simulink model "deadbeat_running_control"  (R2016b)
settings: configuration reference "Configuration1khz" (kept outside this file)
undefined symbols (not defined in the file or in its folder): A_kalman_no_position, A_kalman_transverse, A_kalman_vertical, A_lpf_accelerometer, A_lpf_contact, A_lpf_imu, A_lpf_lateral_angle, B1_lpf_accelerometer, B1_lpf_contact, B1_lpf_imu, B1_lpf_lateral_angle, B2_lpf_accelerometer, B2_lpf_contact, B2_lpf_imu, B2_lpf_lateral_angle, B_dx_versus_x0, B_kalman_no_position, B_kalman_transverse, B_kalman_vertical, backwards_K_sag_of_t, backwards_P_sag_of_t, C_kalman_no_position, C_kalman_transverse, C_kalman_vertical, com_leg_motor, com_torso, contact_threshold, d_ankle_to_foot, d_vertical_com, desired_com_forward_velocity, desired_com_lateral_velocity, desired_standing_torso_pitch, desired_standing_torso_roll, desired_standing_z, desired_torso_pitch, desired_torso_roll, DiscIntNeverNeededParam, Discrete, enable_bouncing, fdesignblkfcn, flight_duration, forward_dx_of_dxstar, forward_x_of_dxstar, g, gcbh, HIP_MTR_MAX_CONT_TORQUE, HIP_MTR_MAX_TORQUE, i_leg_motor, i_robot, i_torso, initial_dx_estimate, initial_dx_takeoff_history, initial_dx_touchdown_history, initial_dy_estimate, initial_dy_takeoff_history, initial_dy_touchdown_history, initial_dz_estimate, initial_leg_selection, initial_target_dx_history, initial_target_dy_history ... (+80)
libraries: simulink x22, ctrlSharedLib x4, dsparch4 x2
(part 5 of 7)

== matlab function deadbeat_running_control/Behavior/Primary and Lateral Behavior/Circular Buffer (Right Foot)/Buffer1 ==
  data: initial_data input; data input; buffer output size=recorded_steps; trigger input; buffer_size input
function buffer  = buffer_data(initial_data, data, trigger, buffer_size)

    persistent buffer_memory
    coder.varsize('buffer_memory',500);
    if isempty(buffer_memory)
        buffer_memory = initial_data;
        if isnan(initial_data(1))
            buffer_memory = [];
        end
    end
    
    if trigger
        buffer_memory = [data; buffer_memory];
        if size(buffer_memory, 1) > buffer_size
            buffer_memory = buffer_memory(1:buffer_size,:);
        end
    end
    
    buffer = buffer_memory;

end

== matlab function deadbeat_running_control/Behavior/Primary and Lateral Behavior/Circular Buffer (Right Foot)/Buffer2 ==
  data: initial_data input; data input; buffer output size=recorded_steps; trigger input; buffer_size input
function buffer  = buffer_data(initial_data, data, trigger, buffer_size)

    persistent buffer_memory
    coder.varsize('buffer_memory',500);
    if isempty(buffer_memory)
        buffer_memory = initial_data;
        if isnan(initial_data(1))
            buffer_memory = [];
        end
    end
    
    if trigger
        buffer_memory = [data; buffer_memory];
        if size(buffer_memory, 1) > buffer_size
            buffer_memory = buffer_memory(1:buffer_size,:);
        end
    end
    
    buffer = buffer_memory;

end

== matlab function deadbeat_running_control/Behavior/Atrias Swing control/Avoid Hitting Mechanical Limits ==
  data: back_cmd output double; front_cmd output double; dback_cmd output double; dfront_cmd output double; ddback_cmd output double; ddfront_cmd output double; back_desired input; dback_desired input; ddback_desired input; front_desired input; dfront_desired input; ddfront_desired input; min_front_bar_angle parameter; max_front_bar_angle parameter; min_back_bar_angle parameter; max_back_bar_angle parameter
%% Avoid joint limits by ensuring we don't command velocities/accelerations that would push us into them when we are close to them.
function [back_cmd, front_cmd, dback_cmd, dfront_cmd, ddback_cmd, ddfront_cmd] ...
    = AvoidFourbarLimits(back_desired,dback_desired, ddback_desired, ...
          front_desired, dfront_desired, ddfront_desired, ...
          min_front_bar_angle, max_front_bar_angle, min_back_bar_angle, max_back_bar_angle)
    [back_cmd, front_cmd, dback_cmd, dfront_cmd, ddback_cmd, ddfront_cmd] = AvoidFourbarLimits(back_desired,dback_desired, ddback_desired, front_desired, dfront_desired, ddfront_desired, min_front_bar_angle, max_front_bar_angle, min_back_bar_angle, max_back_bar_angle);
end

== matlab function deadbeat_running_control/Behavior/Atrias Swing control/Convert COM Position to Joint Angles + Leg Length  ==
  data: desired_leg_length output; X_star input; Y_star input; Z_star input; right_left input; com_pelvis_body input; desired_alpha output; desired_beta output; dcom_pelvis_body input; roll input; pitch input; sagittal_angle input; lateral_angle input; leg_length input; lateral_offset parameter; minimum_lateral_beta parameter; maximum_lateral_beta parameter
function [ desired_leg_length, desired_alpha, desired_beta ]  =  ...
          ConvertToJointAnglesAndLegLength(X_star, Y_star, Z_star, right_left,...
                           com_pelvis_body, dcom_pelvis_body, ...
                           roll, pitch, sagittal_angle, lateral_angle, leg_length,...
                           lateral_offset, minimum_lateral_beta, maximum_lateral_beta) 

    q = [roll(1), pitch(1), sagittal_angle(1), lateral_angle(1), leg_length(1)];
    dq = [roll(2), pitch(2), sagittal_angle(2), lateral_angle(2), leg_length(2)];
    [desired_alpha, desired_beta, desired_leg_length]  =  ConvertComPositionToLegAnglesAndLegLength(X_star, Y_star, Z_star, right_left, com_pelvis_body, dcom_pelvis_body, q, dq, lateral_offset);   
    desired_beta = saturate(desired_beta, minimum_lateral_beta, maximum_lateral_beta);
end

function [desired_saturated] = saturate(desired, minimum_lateral_beta, maximum_lateral_beta)
    desired_saturated = desired;
    if desired(1) < minimum_lateral_beta
        desired_saturated = [minimum_lateral_beta; 0; 0];
    elseif desired(1) > maximum_lateral_beta
        desired_saturated = [maximum_lateral_beta; 0; 0];    
    end
end

== matlab function deadbeat_running_control/Behavior/Atrias Swing control/Virtual Leg to Four Bar ==
  data: l_leg input; dl_leg input; ddl_leg input; phi input; dphi input; ddphi input; back output; dback output; ddback output; front output; dfront output; ddfront output
function [back, dback, ddback, front, dfront, ddfront] = VirtualLegToFourBar(l_leg, dl_leg, ddl_leg, phi, dphi, ddphi)
    [back, dback, ddback, front, dfront, ddfront] = VirtualLegToFourBar(l_leg, dl_leg, ddl_leg, phi, dphi, ddphi);
end

== matlab function deadbeat_running_control/Behavior/Primary and Lateral Behavior/Circular Buffer (Right Foot)/Buffer3 ==
  data: initial_data input; data input; buffer output size=recorded_steps; trigger input; buffer_size input
function buffer  = buffer_data(initial_data, data, trigger, buffer_size)

    persistent buffer_memory
    coder.varsize('buffer_memory',500);
    if isempty(buffer_memory)
        buffer_memory = initial_data;
        if isnan(initial_data(1))
            buffer_memory = [];
        end
    end
    
    if trigger
        buffer_memory = [data; buffer_memory];
        if size(buffer_memory, 1) > buffer_size
            buffer_memory = buffer_memory(1:buffer_size,:);
        end
    end
    
    buffer = buffer_memory;

end

== matlab function deadbeat_running_control/Behavior/Primary and Lateral Behavior/Circular Buffer (Right Foot)/Buffer4 ==
  data: initial_data input; data input; buffer output size=recorded_steps; trigger input; buffer_size input
function buffer  = buffer_data(initial_data, data, trigger, buffer_size)

    persistent buffer_memory
    coder.varsize('buffer_memory',500);
    if isempty(buffer_memory)
        buffer_memory = initial_data;
        if isnan(initial_data(1))
            buffer_memory = [];
        end
    end
    
    if trigger
        buffer_memory = [data; buffer_memory];
        if size(buffer_memory, 1) > buffer_size
            buffer_memory = buffer_memory(1:buffer_size,:);
        end
    end
    
    buffer = buffer_memory;

end

== stateflow chart deadbeat_running_control/Behavior/Contact State Machine/State Machine ==
  state Touchdown
  state Unloading
  state Takeoff
  state Flight
  Touchdown -> (junction 162) [order 2] : [contact_factor < 0.5*contact_threshold]
  (junction 162) -> (junction 128)
  (junction 115) -> Touchdown
  (junction 118) -> (junction 115)
  Touchdown -> Unloading [order 1] : [z_velocity >= 0 && previous_z_velocity < 0]
  Unloading -> Touchdown [order 2] : [contact_factor > contact_threshold && z_velocity < 0]
  (junction 122) -> (junction 118)
  Unloading -> Takeoff [order 1] : [contact_factor < contact_threshold]
  (junction 172) -> (junction 122)
  Takeoff -> Flight : after(t_flight,sec)
  (default) -> Flight
  Flight -> (junction 172) : [contact_factor > variable_contact_threshold]
  (junction 128) -> Flight
  data: z_velocity input; previous_z_velocity input; contact_factor input; t_flight parameter; contact_threshold parameter; Touchdown output boolean; Unloading output boolean; Takeoff output boolean; Flight output boolean; variable_contact_threshold input

== matlab function deadbeat_running_control/Behavior/Primary and Lateral Behavior/Circular Buffer (Right Foot)/Buffer6 ==
  data: initial_data input; data input; buffer output size=recorded_steps; trigger input; buffer_size input
function buffer  = buffer_data(initial_data, data, trigger, buffer_size)

    persistent buffer_memory
    coder.varsize('buffer_memory',500);
    if isempty(buffer_memory)
        buffer_memory = initial_data;
        if isnan(initial_data(1))
            buffer_memory = [];
        end
    end
    
    if trigger
        buffer_memory = [data; buffer_memory];
        if size(buffer_memory, 1) > buffer_size
            buffer_memory = buffer_memory(1:buffer_size,:);
        end
    end
    
    buffer = buffer_memory;

end

== matlab function deadbeat_running_control/Behavior/Force Estimation/3D Forward Dynamics yawed ==
  data: right_or_left input; torso_roll input size=2; torso_pitch input double size=2; torso_yaw input double size=2; primary_sagittal_leg_angle input double size=2; primary_leg_length input double size=2; primary_leg_roll input double size=2; secondary_leg_roll input double size=2; primary_leg_torque input; primary_leg_force input; primary_lateral_torque input; secondary_lateral_torque input; R_GRF output double size=3; L_GRF output size=3; ddroll output double; g parameter; m_leg_motor parameter; m_torso parameter; i_torso parameter; i_leg_motor parameter; lateral_offset parameter; com_torso parameter; torso_centerline_roll_offset_angle parameter
%% Forward 3D ATRIAS dynamics
function [R_GRF, L_GRF, ddroll]  =  ForwardDynamics3D(right_or_left, ...
                                                      torso_roll, torso_pitch, torso_yaw, ...
                                                      primary_sagittal_leg_angle, primary_leg_length,...
                                                      primary_leg_roll, secondary_leg_roll, ...
                                                      primary_leg_torque, primary_leg_force, ...
                                                      primary_lateral_torque, secondary_lateral_torque, ...
                                                      g, m_leg_motor, m_torso, i_torso, i_leg_motor, lateral_offset, com_torso, torso_centerline_roll_offset_angle)

    d = norm(com_torso(2:3));
    It = mean(i_torso);
    Im = mean(i_leg_motor);
    
    phi    = torso_roll(1) + torso_centerline_roll_offset_angle;  % roll
    theta  = torso_pitch(1);                   % pitch
    alpha1 = primary_sagittal_leg_angle(1);    % primary sagittal leg angle
    beta1  = primary_leg_roll(1);              % primary leg roll
    beta2  = secondary_leg_roll(1);            % secondary leg roll
    if right_or_left
        beta1 = beta1 - torso_centerline_roll_offset_angle;
        beta2 = beta2 + torso_centerline_roll_offset_angle;
    else
        beta1 = beta1 + torso_centerline_roll_offset_angle;
        beta2 = beta2 - torso_centerline_roll_offset_angle;
    end 
    l1     = primary_leg_length(1);            % primary leg length
    
    dphi    = torso_roll(2);
    dtheta  = torso_pitch(2);
    dpsi    = torso_yaw(2);
    dalpha1 = primary_sagittal_leg_angle(2);
    dbeta1  = primary_leg_roll(2);
    dbeta2  = secondary_leg_roll(2);
    dl1     = primary_leg_length(2);
    
    
    tau_a1 = primary_leg_torque;
    tau_b1 = primary_lateral_torque;
    tau_b2 = secondary_lateral_torque;
    F_l1 = primary_leg_force;

    if right_or_left == 1
      A = A_fwd_yawed_right(lateral_offset,d,m_leg_motor,m_torso,It,Im,phi,theta,alpha1,beta1,beta2,l1);
      B = B_fwd_yawed_right(lateral_offset,d,g,m_leg_motor,m_torso,It,Im,phi,theta,alpha1,beta1,beta2,l1,dphi,dtheta,dpsi,dalpha1,dbeta1,dbeta2,dl1,tau_a1,tau_b1,tau_b2,F_l1);
    else
      A = A_fwd_yawed_left(lateral_offset,d,m_leg_motor,m_torso,It,Im,phi,theta,alpha1,beta1,beta2,l1);
      B = B_fwd_yawed_left(lateral_offset,d,g,m_leg_motor,m_torso,It,Im,phi,theta,alpha1,beta1,beta2,l1,dphi,dtheta,dpsi,dalpha1,dbeta1,dbeta2,dl1,tau_a1,tau_b1,tau_b2,F_l1);
    end
    
    x_fwd = A \ B;
    ddroll = x_fwd(4);
    GRF = zeros(3,1);
    GRF(1) = x_fwd(11);
    GRF(2) = x_fwd(12);
    GRF(3) = x_fwd(13); 
    
    if right_or_left == 1
        R_GRF = GRF;
        L_GRF = [0;0;0];
    else
        R_GRF = [0;0;0];
        L_GRF = GRF;
    end
end

== matlab function deadbeat_running_control/Behavior/Force Estimation/Leg Force Measurements/Nonlinear Spring Force ==
  data: deflections input; tau_sea output
function tau_sea   = SeaSpringForce( deflections )
    tau_sea = SeaSpringForce( deflections );
end

== matlab function deadbeat_running_control/Behavior/Knee Torques ==
  data: right_knees_to_foot input; right_front_knee_torques_from_fd output; left_knees_to_foot input; grf_from_seas input; grf_from_accelerometer input; right_back_knee_torques_from_fd output; right_front_knee_torques_from_accelerometer output; right_back_knee_torques_from_accelerometer output; left_front_knee_torques_from_fd output; left_back_knee_torques_from_fd output; left_front_knee_torques_from_accelerometer output; left_back_knee_torques_from_accelerometer output
function [right_front_knee_torques_from_fd, right_back_knee_torques_from_fd,...
          right_front_knee_torques_from_accelerometer, right_back_knee_torques_from_accelerometer,...
          left_front_knee_torques_from_fd, left_back_knee_torques_from_fd,...
          left_front_knee_torques_from_accelerometer, left_back_knee_torques_from_accelerometer] ...
          = compute_knee_torques(right_knees_to_foot, left_knees_to_foot, grf_from_seas, grf_from_accelerometer)

      right_front_knee_torques_from_fd = cross(right_knees_to_foot(1:3), grf_from_seas);
      right_back_knee_torques_from_fd = cross(right_knees_to_foot(4:6), grf_from_seas);
      right_front_knee_torques_from_accelerometer = cross(right_knees_to_foot(1:3), grf_from_accelerometer);
      right_back_knee_torques_from_accelerometer = cross(right_knees_to_foot(4:6), grf_from_accelerometer);
      
      left_front_knee_torques_from_fd = cross(left_knees_to_foot(1:3), grf_from_seas);
      left_back_knee_torques_from_fd = cross(left_knees_to_foot(4:6), grf_from_seas);
      left_front_knee_torques_from_accelerometer = cross(left_knees_to_foot(1:3), grf_from_accelerometer);
      left_back_knee_torques_from_accelerometer = cross(left_knees_to_foot(4:6), grf_from_accelerometer);
end

== matlab function deadbeat_running_control/Behavior/Primary Secondary Leg Swap/ToggleRightLeftLeg ==
  data: toggle input boolean; right_left output double; previous_right_left input double
function right_left = ToggleRightLeftLeg(toggle, previous_right_left)
    
    if toggle
        right_left = -previous_right_left + 1;
    else
        right_left = previous_right_left;
    end

end

== matlab function deadbeat_running_control/Behavior/Primary and Lateral Behavior/Circular Buffer (Right Foot)/Buffer7 ==
  data: initial_data input; data input; buffer output size=recorded_steps; trigger input; buffer_size input
function buffer  = buffer_data(initial_data, data, trigger, buffer_size)

    persistent buffer_memory
    coder.varsize('buffer_memory',500);
    if isempty(buffer_memory)
        buffer_memory = initial_data;
        if isnan(initial_data(1))
            buffer_memory = [];
        end
    end
    
    if trigger
        buffer_memory = [data; buffer_memory];
        if size(buffer_memory, 1) > buffer_size
            buffer_memory = buffer_memory(1:buffer_size,:);
        end
    end
    
    buffer = buffer_memory;

end

== matlab function deadbeat_running_control/Behavior/Primary and Lateral Behavior/Circular Buffer (Right Foot)/Buffer8 ==
  data: initial_data input; data input; buffer output size=recorded_steps; trigger input; buffer_size input
function buffer  = buffer_data(initial_data, data, trigger, buffer_size)

    persistent buffer_memory
    coder.varsize('buffer_memory',500);
    if isempty(buffer_memory)
        buffer_memory = initial_data;
        if isnan(initial_data(1))
            buffer_memory = [];
        end
    end
    
    if trigger
        buffer_memory = [data; buffer_memory];
        if size(buffer_memory, 1) > buffer_size
            buffer_memory = buffer_memory(1:buffer_size,:);
        end
    end
    
    buffer = buffer_memory;

end

== matlab function deadbeat_running_control/Behavior/Primary and Lateral Behavior/Buffer5 ==
  data: data input; trigger input; average output
function average  = average_data(data, trigger)

    persistent buffer_memory
    coder.varsize('buffer_memory',20);
    if isempty(buffer_memory)
        buffer_memory = 0;
    end

    if trigger
        buffer_size = 4;
        buffer_memory = [data; buffer_memory];
        if size(buffer_memory, 1) > buffer_size
            buffer_memory = buffer_memory(1:buffer_size,:);
        end
    end
    
    average = mean(buffer_memory);

end

== matlab function deadbeat_running_control/Behavior/Primary and Lateral Behavior/Circular Buffer (Left Foot)/Buffer1 ==
  data: initial_data input; data input; buffer output size=recorded_steps; trigger input; buffer_size input
function buffer  = buffer_data(initial_data, data, trigger, buffer_size)

    persistent buffer_memory
    coder.varsize('buffer_memory',500);
    if isempty(buffer_memory)
        buffer_memory = initial_data;
        if isnan(initial_data(1))
            buffer_memory = [];
        end
    end
    
    if trigger
        buffer_memory = [data; buffer_memory];
        if size(buffer_memory, 1) > buffer_size
            buffer_memory = buffer_memory(1:buffer_size,:);
        end
    end
    
    buffer = buffer_memory;

end

== matlab function deadbeat_running_control/Behavior/Primary and Lateral Behavior/Circular Buffer (Left Foot)/Buffer2 ==
  data: initial_data input; data input; buffer output size=recorded_steps; trigger input; buffer_size input
function buffer  = buffer_data(initial_data, data, trigger, buffer_size)

    persistent buffer_memory
    coder.varsize('buffer_memory',500);
    if isempty(buffer_memory)
        buffer_memory = initial_data;
        if isnan(initial_data(1))
            buffer_memory = [];
        end
    end
    
    if trigger
        buffer_memory = [data; buffer_memory];
        if size(buffer_memory, 1) > buffer_size
            buffer_memory = buffer_memory(1:buffer_size,:);
        end
    end
    
    buffer = buffer_memory;

end

== matlab function deadbeat_running_control/Behavior/Primary and Lateral Behavior/Circular Buffer (Left Foot)/Buffer3 ==
  data: initial_data input; data input; buffer output size=recorded_steps; trigger input; buffer_size input
function buffer  = buffer_data(initial_data, data, trigger, buffer_size)

    persistent buffer_memory
    coder.varsize('buffer_memory',500);
    if isempty(buffer_memory)
        buffer_memory = initial_data;
        if isnan(initial_data(1))
            buffer_memory = [];
        end
    end
    
    if trigger
        buffer_memory = [data; buffer_memory];
        if size(buffer_memory, 1) > buffer_size
            buffer_memory = buffer_memory(1:buffer_size,:);
        end
    end
    
    buffer = buffer_memory;

end

== matlab function deadbeat_running_control/Behavior/Primary and Lateral Behavior/Circular Buffer (Left Foot)/Buffer4 ==
  data: initial_data input; data input; buffer output size=recorded_steps; trigger input; buffer_size input
function buffer  = buffer_data(initial_data, data, trigger, buffer_size)

    persistent buffer_memory
    coder.varsize('buffer_memory',500);
    if isempty(buffer_memory)
        buffer_memory = initial_data;
        if isnan(initial_data(1))
            buffer_memory = [];
        end
    end
    
    if trigger
        buffer_memory = [data; buffer_memory];
        if size(buffer_memory, 1) > buffer_size
            buffer_memory = buffer_memory(1:buffer_size,:);
        end
    end
    
    buffer = buffer_memory;

end

== matlab function deadbeat_running_control/Behavior/Primary and Lateral Behavior/Circular Buffer (Left Foot)/Buffer5 ==
  data: initial_data input; data input; buffer output size=recorded_steps; trigger input; buffer_size input
function buffer  = buffer_data(initial_data, data, trigger, buffer_size)

    persistent buffer_memory
    coder.varsize('buffer_memory',500);
    if isempty(buffer_memory)
        buffer_memory = initial_data;
        if isnan(initial_data(1))
            buffer_memory = [];
        end
    end
    
    if trigger
        buffer_memory = [data; buffer_memory];
        if size(buffer_memory, 1) > buffer_size
            buffer_memory = buffer_memory(1:buffer_size,:);
        end
    end
    
    buffer = buffer_memory;

end

== matlab function deadbeat_running_control/Behavior/Primary and Lateral Behavior/Circular Buffer (Left Foot)/Buffer6 ==
  data: initial_data input; data input; buffer output size=recorded_steps; trigger input; buffer_size input
function buffer  = buffer_data(initial_data, data, trigger, buffer_size)

    persistent buffer_memory
    coder.varsize('buffer_memory',500);
    if isempty(buffer_memory)
        buffer_memory = initial_data;
        if isnan(initial_data(1))
            buffer_memory = [];
        end
    end
    
    if trigger
        buffer_memory = [data; buffer_memory];
        if size(buffer_memory, 1) > buffer_size
            buffer_memory = buffer_memory(1:buffer_size,:);
        end
    end
    
    buffer = buffer_memory;

end

== matlab function deadbeat_running_control/Behavior/Primary and Lateral Behavior/Circular Buffer (Left Foot)/Buffer7 ==
  data: initial_data input; data input; buffer output size=recorded_steps; trigger input; buffer_size input
function buffer  = buffer_data(initial_data, data, trigger, buffer_size)

    persistent buffer_memory
    coder.varsize('buffer_memory',500);
    if isempty(buffer_memory)
        buffer_memory = initial_data;
        if isnan(initial_data(1))
            buffer_memory = [];
        end
    end
    
    if trigger
        buffer_memory = [data; buffer_memory];
        if size(buffer_memory, 1) > buffer_size
            buffer_memory = buffer_memory(1:buffer_size,:);
        end
    end
    
    buffer = buffer_memory;

end

== matlab function deadbeat_running_control/Behavior/Primary and Lateral Behavior/Circular Buffer (Left Foot)/Buffer8 ==
  data: initial_data input; data input; buffer output size=recorded_steps; trigger input; buffer_size input
function buffer  = buffer_data(initial_data, data, trigger, buffer_size)

    persistent buffer_memory
    coder.varsize('buffer_memory',500);
    if isempty(buffer_memory)
        buffer_memory = initial_data;
        if isnan(initial_data(1))
            buffer_memory = [];
        end
    end
    
    if trigger
        buffer_memory = [data; buffer_memory];
        if size(buffer_memory, 1) > buffer_size
            buffer_memory = buffer_memory(1:buffer_size,:);
        end
    end
    
    buffer = buffer_memory;

end

== matlab function deadbeat_running_control/Behavior/Primary and Lateral Behavior/Closed Loop Compensation (Left Foot)/CLOSED LOOP COMPENSATION X FOR VAIRABLE SPEED ==
  data: A_cl input; epsilon input; c input; delta_s_i input; dx_star input; B_cl input; delta_ux output
function delta_ux  = closed_loop_compensation_dxstar...
         (A_cl,epsilon, c, delta_s_i, dx_star, B_cl)
% assume form of delta_s_{i+1} = A_cl*delta_s_i + epsilon +c*dx_star + B_cl*delta_ux
% where delta measures deviation from deadbeat case. solve for
% delta_ux = (-A_cl*delta_s_i-epsilon - c*dxstar)/B_cl to achieve deadbeat
delta_ux = (-A_cl*delta_s_i - epsilon - c*dx_star)/B_cl;

== matlab function deadbeat_running_control/Behavior/Primary and Lateral Behavior/Closed Loop Compensation (Left Foot)/CLOSED LOOP COMPENSATION Y FOR VAIRABLE SPEED ==
  data: A_cl input; epsilon input; c input; delta_s_i input; dx_star input; B_cl input; delta_ux output
function delta_ux  = closed_loop_compensation_dxstar...
         (A_cl,epsilon, c, delta_s_i, dx_star, B_cl)
% assume form of delta_s_{i+1} = A_cl*delta_s_i + epsilon +c*dx_star + B_cl*delta_ux
% where delta measures deviation from deadbeat case. solve for
% delta_ux = (-A_cl*delta_s_i-epsilon - c*dxstar)/B_cl to achieve deadbeat
delta_ux = (-A_cl*delta_s_i - epsilon - c*dx_star)/B_cl;

== matlab function deadbeat_running_control/Behavior/Primary and Lateral Behavior/Closed Loop Compensation (Left Foot)/ESTIMATE CLOSED LOOP ERROR X FOR VARIABLE SPEED ==
  data: dx_land_hist input; A_cl output; delta_ux_hist input; dx_lift_hist input; dx_star_hist input; B_dx_versus_x0 parameter; W_real input; epsilon_0 output; c output; A_cl_nb output; epsilon_0_nb output; c_nb output
function [A_cl, epsilon_0, c, ...
          A_cl_nb, epsilon_0_nb, c_nb] = error_fitting_dxstar...
         (dx_land_hist, delta_ux_hist, dx_lift_hist, dx_star_hist,...
          B_dx_versus_x0, W_real)
% data_length = min([length(dx_lift_hist), filter_length]);
data_length = length(dx_lift_hist);
assert(data_length < 500);
% add fake data
fake_dx_land_err_magnitude = 0.1; fake_dx_star_magnitude = 0.1;
[fgrid_dx_land_err, fgrid_dx_star, fgrid_dx_lift_err] = ...
    meshgrid(fake_dx_land_err_magnitude*[-1 1],fake_dx_star_magnitude*[-1 1],0);
fake_data_length = numel(fgrid_dx_land_err);
fake_dx_land_err = fgrid_dx_land_err(:);
fake_dx_star = fgrid_dx_star(:);
fake_dx_lift_err = fgrid_dx_lift_err(:);
fake_delta_ux = zeros(fake_data_length,1);
% assert(fake_data_length<100);
% assert(filter_length<100);
% fake_dx_land_err = linspace(-0.1, 0.1, fake_data_length)';
% fake_dx_lift_err = zeros(fake_data_length,1);
% fake_delta_ux = zeros(fake_data_length,1);
% fake_dx_star = linspace(-0.25, 0.25, fake_data_length)';
dx_land_err = [reshape(dx_land_hist(1:data_length)-dx_star_hist(1:data_length),...
                       data_length, 1); fake_dx_land_err];
dx_lift_err = [reshape(dx_lift_hist(1:data_length)-dx_star_hist(1:data_length),...
                       data_length, 1); fake_dx_lift_err];
dx_star = [reshape(dx_star_hist(1:data_length), data_length,1); fake_dx_star];
delta_ux = [reshape(delta_ux_hist(1:data_length), data_length, 1); fake_delta_ux];
% weighted least squares
W = diag([W_real*ones(1,data_length), ones(1,fake_data_length)]);
Y = dx_lift_err - B_dx_versus_x0*delta_ux;
X = [dx_land_err, dx_star, ones(data_length+fake_data_length,1)];
% linear regression for s_{i+1}-s0 = A_cl*(s_i-s0) + epsilon_0 + c(s0) + B*delta_u
% solve for Y = X*beta, beta column vector
beta_hat = (X'*W*X)\X'*W*Y;
W_nobias = diag([W_real*ones(1,data_length), 0.001*ones(1,fake_data_length)]);
beta_hat_nobias = (X'*W_nobias*X)\X'*W_nobias*Y;
A_cl = beta_hat(1);
c = beta_hat(2);
epsilon_0 = beta_hat(3);
A_cl_nb = beta_hat_nobias(1);
c_nb = beta_hat_nobias(2);
epsilon_0_nb = beta_hat_nobias(3);

== matlab function deadbeat_running_control/Behavior/Atrias Swing control/Avoid Virtual Leg Length Limits ==
  data: l_leg_desired input; dl_leg_desired input; ddl_leg_desired input; l_leg_cmd output double; dl_leg_cmd output double; ddl_leg_cmd output double; min_leg_length parameter; max_leg_length parameter
%% Avoid virtual leg length limits by ensuring we don't command position/velocities/accelerations that would hit them.
function [l_leg_cmd, dl_leg_cmd, ddl_leg_cmd] = AvoidVirtualLengthLimits(l_leg_desired, dl_leg_desired, ddl_leg_desired, min_leg_length, max_leg_length)
    [l_leg_cmd, dl_leg_cmd, ddl_leg_cmd] = AvoidVirtualLengthLimits(l_leg_desired, dl_leg_desired, ddl_leg_desired, min_leg_length, max_leg_length);
end

== matlab function deadbeat_running_control/Behavior/Primary and Lateral Behavior/Closed Loop Compensation (Left Foot)/ESTIMATE CLOSED LOOP ERROR Y FOR VARIABLE SPEED ==
  data: dx_land_hist input; A_cl output; delta_ux_hist input; dx_lift_hist input; dx_star_hist input; B_dx_versus_x0 parameter; W_real input; epsilon_0 output; c output; A_cl_nb output; epsilon_0_nb output; c_nb output
function [A_cl, epsilon_0, c, ...
          A_cl_nb, epsilon_0_nb, c_nb] = error_fitting_dxstar...
         (dx_land_hist, delta_ux_hist, dx_lift_hist, dx_star_hist,...
          B_dx_versus_x0, W_real)
% data_length = min([length(dx_lift_hist), filter_length]);
data_length = length(dx_lift_hist);
assert(data_length < 500);
% add fake data
fake_dx_land_err_magnitude = 0.1; fake_dx_star_magnitude = 0.1;
[fgrid_dx_land_err, fgrid_dx_star, fgrid_dx_lift_err] = ...
    meshgrid(fake_dx_land_err_magnitude*[-1 1],fake_dx_star_magnitude*[-1 1],0);
fake_data_length = numel(fgrid_dx_land_err);
fake_dx_land_err = fgrid_dx_land_err(:);
fake_dx_star = fgrid_dx_star(:);
fake_dx_lift_err = fgrid_dx_lift_err(:);
fake_delta_ux = zeros(fake_data_length,1);
% assert(fake_data_length<100);
% assert(filter_length<100);
% fake_dx_land_err = linspace(-0.1, 0.1, fake_data_length)';
% fake_dx_lift_err = zeros(fake_data_length,1);
% fake_delta_ux = zeros(fake_data_length,1);
% fake_dx_star = linspace(-0.25, 0.25, fake_data_length)';
dx_land_err = [reshape(dx_land_hist(1:data_length)-dx_star_hist(1:data_length),...
                       data_length, 1); fake_dx_land_err];
dx_lift_err = [reshape(dx_lift_hist(1:data_length)-dx_star_hist(1:data_length),...
                       data_length, 1); fake_dx_lift_err];
dx_star = [reshape(dx_star_hist(1:data_length), data_length,1); fake_dx_star];
delta_ux = [reshape(delta_ux_hist(1:data_length), data_length, 1); fake_delta_ux];
% weighted least squares
W = diag([W_real*ones(1,data_length), ones(1,fake_data_length)]);
Y = dx_lift_err - B_dx_versus_x0*delta_ux;
X = [dx_land_err, dx_star, ones(data_length+fake_data_length,1)];
% linear regression for s_{i+1}-s0 = A_cl*(s_i-s0) + epsilon_0 + c(s0) + B*delta_u
% solve for Y = X*beta, beta column vector
beta_hat = (X'*W*X)\X'*W*Y;
W_nobias = diag([W_real*ones(1,data_length), 0.001*ones(1,fake_data_length)]);
beta_hat_nobias = (X'*W_nobias*X)\X'*W_nobias*Y;
A_cl = beta_hat(1);
c = beta_hat(2);
epsilon_0 = beta_hat(3);
A_cl_nb = beta_hat_nobias(1);
c_nb = beta_hat_nobias(2);
epsilon_0_nb = beta_hat_nobias(3);

== matlab function deadbeat_running_control/Behavior/Primary and Lateral Behavior/Desired Forward Velocity1 ==
  data: step_count input; desired_dx output; forward_velocity_nominal_gait parameter; stop_running output boolean; stop_controller output
function [desired_dx, stop_running, stop_controller] = dx_command(step_count, forward_velocity_nominal_gait)

    desired_dx = 0;
    if step_count <= length(forward_velocity_nominal_gait) && step_count >= 1
        desired_dx = forward_velocity_nominal_gait(step_count);
    end
    
    stop_running = false;
    stop_controller = false;
    if step_count > length(forward_velocity_nominal_gait) + 1
        stop_running = true;
    end
    if step_count > length(forward_velocity_nominal_gait) + 2
        stop_controller = true;
    end

end

== matlab function deadbeat_running_control/Behavior/Primary and Lateral Behavior/Stance/2D Inverse Dynamics/target_GRF_inverse_dynamics ==
  data: GRFx input; GRFz input; z output; theta input; phi input; l_leg input; w input; tau_rotor_f input; tau_rotor_b input; d_vertical_com parameter; LEG_MTR_GEAR_RATIO parameter; g parameter; j_leg parameter; i_robot parameter; m_total_real parameter; m_leg parameter
%% Inverse dynamics
% Inputs:  gamma, dgamma, theta, dtheta,  GRFx_des, GRFy_des
% Outputs: ddx,   ddy,    ddl,   ddgamma, ddtheta,  tau_sf,  tau_sb
function z = fcn(GRFx, GRFz, theta, phi, l_leg, w,...
                                  tau_rotor_f, tau_rotor_b, ...
                                  d_vertical_com, LEG_MTR_GEAR_RATIO, g,...
                                  j_leg, i_robot, ...
                                  m_total_real, m_leg)
              
    % Parameters
    m      = m_total_real;    % mass of system + boom
    Il     = j_leg;             % inertia of leg
    It     = i_robot;           % inertia of system3.
    d      = d_vertical_com;             % distance from hip to system COM
    g1     = phi(1)+theta(1);   % global leg angle (after spring)
    dg1    = phi(2)+theta(2);
    th     = theta(1);          % global torso angle   
    dth    = theta(2);
    t_rf   = tau_rotor_f;       % torque applied at front rotor 
    t_rb   = tau_rotor_b;       % torque applied at back rotor
    N      = -LEG_MTR_GEAR_RATIO;
    l      = l_leg(1);          % leg length
    dl     = l_leg(2);
    
    % Stance dynamics (P z = [h; -dJ*dq] + [J zeros(2,2)]^T F)
    %     J  = [1  0  sin(g1)     l*cos(g1)   -d*cos(th);
    %           0  1  cos(g1)    -l*sin(g1)    d*sin(th)];
    %       
    %     dJ = [0  0   dg1*cos(g1)    (-l*dg1*sin(g1)+dl*cos(g1))  d*dth*sin(th);
    %           0  0  -dg1*sin(g1)    (-1*dg1*cos(g1)-dl*sin(g1))  d*dth*cos(th)];
    % 
    %     dq  = [dx  dz  dl  dg1  dth ]';
    %       
    %     M = [m  0   0       0    0; 
    %          0  m   0       0    0;
    %          0  0   m_leg   0    0;   
    %          0  0   0       Il   0;  
    %          0  0   0       0    It];  
    %     
    %     h = [0; -m*g_reduced; 0; 0; (-t_rf-t_rb)];
    % 
    %     S = [ 0         0;
    %           0         0;
    %           1/w      -1/w;
    %           1         1;
    %          -(N-1)/N  -(N-1)/N];
    % 
    %     F = [GRFx GRFz]';
    %     
    %     P = [M              -S;       
    %          J               zeros(2,2)];
    
    % Solving for z:    
    %     ddq = [ddx ddy ddl ddg1 ddth]';
    %     z = [ddq; t_sf; t_sb];
    %     z = P\([h; -dJ*dq] + [J zeros(2,2)]'*F);
    
    z =  [GRFx/m;
         (GRFz - g*m)/m;
        -(Il*d*dg1^2*m*cos(g1 - th) - 2*GRFx*Il*d*sin(th) - 2*Il*d^2*dth^2*m - GRFz*d*l^2*m*cos(th) - GRFx*d*l^2*m*sin(th) - 2*GRFz*Il*d*cos(th) + 2*GRFz*It*N*l*cos(g1) + 2*GRFz*Il*N*d*cos(th) + 2*GRFx*It*N*l*sin(g1) + 2*GRFx*Il*N*d*sin(th) - It*N*dg1^2*l*m + GRFz*d*l^2*m*cos(2*g1 - th) + GRFx*d*l^2*m*sin(2*g1 - th) + 2*Il*d*g*m*cos(th) + Il*d*dg1^2*m*cos(g1 + th) + 2*Il*N*d^2*dth^2*m - It*N*dg1^2*l^2*m - 2*It*N*g*l*m*cos(g1) - 2*Il*N*d*g*m*cos(th) + It*N*dg1^2*l^2*m*cos(2*g1) - Il*N*d*dg1^2*m*cos(g1 + th) - Il*d*dg1^2*l*m*cos(g1 + th) + 4*Il*d*dg1*dl*m*sin(g1 - th) + GRFz*N*d^2*l*m*cos(g1) + GRFz*N*d*l^2*m*cos(th) + GRFx*N*d^2*l*m*sin(g1) + 2*N*d*l*m*t_rb*sin(g1 - th) + 2*N*d*l*m*t_rf*sin(g1 - th) + GRFx*N*d*l^2*m*sin(th) - Il*N*d*dg1^2*m*cos(g1 - th) - GRFz*N*d^2*l*m*cos(g1 - 2*th) + GRFx*N*d^2*l*m*sin(g1 - 2*th) + Il*d*dg1^2*l*m*cos(g1 - th) - It*N*dg1^2*l*m*cos(2*g1) - GRFz*N*d*l^2*m*cos(2*g1 - th) - GRFx*N*d*l^2*m*sin(2*g1 - th) + Il*N*d*dg1^2*l*m*cos(g1 + th) - 4*Il*N*d*dg1*dl*m*sin(g1 - th) - Il*N*d*dg1^2*l*m*cos(g1 - th) + 2*It*N*d*dth^2*l*m*cos(g1 - th))/(2*m*(It*N*l - Il*d*cos(g1 - th) + Il*N*d*cos(g1 - th)));
        -(2*GRFx*It*N*cos(g1) - 2*GRFz*It*N*sin(g1) + GRFx*N*d^2*m*cos(g1 - 2*th) + 4*It*N*dg1*dl*m + GRFz*N*d^2*m*sin(g1 - 2*th) + GRFx*d*l*m*cos(2*g1 - th) - GRFz*d*l*m*sin(2*g1 - th) + It*N*dg1^2*m*sin(2*g1) + 2*It*N*g*m*sin(g1) + GRFx*d*l*m*cos(th) - GRFz*d*l*m*sin(th) + GRFx*N*d^2*m*cos(g1) + 2*N*d*m*t_rb*cos(g1 - th) + 2*N*d*m*t_rf*cos(g1 - th) - GRFz*N*d^2*m*sin(g1) - GRFx*N*d*l*m*cos(th) + GRFz*N*d*l*m*sin(th) - GRFx*N*d*l*m*cos(2*g1 - th) - 2*It*N*d*dth^2*m*sin(g1 - th) + GRFz*N*d*l*m*sin(2*g1 - th) - It*N*dg1^2*l*m*sin(2*g1))/(2*m*(It*N*l - Il*d*cos(g1 - th) + Il*N*d*cos(g1 - th)));
        -(GRFx*Il*cos(g1) - GRFz*Il*sin(g1) - GRFx*Il*N*cos(g1) + (Il*dg1^2*m*sin(2*g1))/2 + GRFz*Il*N*sin(g1) + Il*g*m*sin(g1) + GRFx*l^2*m*cos(g1) - GRFz*l^2*m*sin(g1) + 2*Il*dg1*dl*m + N*l*m*t_rb + N*l*m*t_rf + GRFz*N*l^2*m*sin(g1) - 2*Il*N*dg1*dl*m - Il*d*dth^2*m*sin(g1 - th) - (Il*N*dg1^2*m*sin(2*g1))/2 - (Il*dg1^2*l*m*sin(2*g1))/2 - Il*N*g*m*sin(g1) - GRFx*N*l^2*m*cos(g1) + GRFx*N*d*l*m*cos(th) - GRFz*N*d*l*m*sin(th) + Il*N*d*dth^2*m*sin(g1 - th) + (Il*N*dg1^2*l*m*sin(2*g1))/2)/(m*(It*N*l - Il*d*cos(g1 - th) + Il*N*d*cos(g1 - th)));
        -(2*GRFx*Il*It*N*cos(g1) - 2*GRFz*Il*It*N*sin(g1) - GRFz*Il*d*m*w*cos(th) - 2*GRFz*Il*d*m_leg*w*cos(th) - GRFx*Il*d*m*w*sin(th) - 2*GRFx*Il*d*m_leg*w*sin(th) + GRFx*Il*N*d^2*m*cos(g1) + 2*Il*N*d*m*t_rb*cos(g1 - th) + 2*Il*N*d*m*t_rf*cos(g1 - th) + 2*GRFx*It*N*l^2*m*cos(g1) - GRFz*Il*N*d^2*m*sin(g1) - 2*GRFz*It*N*l^2*m*sin(g1) + GRFx*Il*N*d^2*m*cos(g1 - 2*th) + 4*Il*It*N*dg1*dl*m + GRFz*Il*N*d^2*m*sin(g1 - 2*th) - 2*Il*d^2*dth^2*m*m_leg*w - GRFz*Il*d*m*w*cos(2*g1 - th) - GRFx*Il*d*m*w*sin(2*g1 - th) + Il*It*N*dg1^2*m*sin(2*g1) + 2*Il*It*N*g*m*sin(g1) - GRFx*d*l^2*m*m_leg*w*sin(th) - Il*It*N*dg1^2*l*m*sin(2*g1) + Il*d*dg1^2*m*m_leg*w*cos(g1 - th) + 2*GRFz*It*N*l*m*w*cos(g1) + 2*GRFz*It*N*l*m_leg*w*cos(g1) + GRFz*Il*N*d*m*w*cos(th) + 2*GRFz*Il*N*d*m_leg*w*cos(th) + 2*GRFx*It*N*l*m*w*sin(g1) + 2*GRFx*It*N*l*m_leg*w*sin(g1) + GRFx*Il*N*d*m*w*sin(th) + 2*GRFx*Il*N*d*m_leg*w*sin(th) - It*N*dg1^2*l*m*m_leg*w + GRFz*d*l^2*m*m_leg*w*cos(2*g1 - th) + GRFx*d*l^2*m*m_leg*w*sin(2*g1 - th) + 2*Il*d*g*m*m_leg*w*cos(th) + Il*d*dg1^2*m*m_leg*w*cos(g1 + th) + 2*Il*N*d^2*dth^2*m*m_leg*w - It*N*dg1^2*l^2*m*m_leg*w - 2*Il*It*N*d*dth^2*m*sin(g1 - th) + GRFz*Il*N*d*m*w*cos(2*g1 - th) + GRFx*Il*N*d*m*w*sin(2*g1 - th) - GRFz*d*l^2*m*m_leg*w*cos(th) + It*N*dg1^2*l^2*m*m_leg*w*cos(2*g1) - Il*N*d*dg1^2*m*m_leg*w*cos(g1 + th) - Il*d*dg1^2*l*m*m_leg*w*cos(g1 + th) + 4*Il*d*dg1*dl*m*m_leg*w*sin(g1 - th) + GRFz*N*d^2*l*m*m_leg*w*cos(g1) + GRFz*N*d*l^2*m*m_leg*w*cos(th) + GRFx*N*d^2*l*m*m_leg*w*sin(g1) + 2*N*d*l*m*m_leg*t_rb*w*sin(g1 - th) + 2*N*d*l*m*m_leg*t_rf*w*sin(g1 - th) + GRFx*N*d*l^2*m*m_leg*w*sin(th) - Il*N*d*dg1^2*m*m_leg*w*cos(g1 - th) - GRFz*N*d^2*l*m*m_leg*w*cos(g1 - 2*th) + GRFx*N*d^2*l*m*m_leg*w*sin(g1 - 2*th) + Il*d*dg1^2*l*m*m_leg*w*cos(g1 - th) - It*N*dg1^2*l*m*m_leg*w*cos(2*g1) - GRFz*N*d*l^2*m*m_leg*w*cos(2*g1 - th) - GRFx*N*d*l^2*m*m_leg*w*sin(2*g1 - th) - 2*It*N*g*l*m*m_leg*w*cos(g1) - 2*Il*N*d*g*m*m_leg*w*cos(th) + Il*N*d*dg1^2*l*m*m_leg*w*cos(g1 + th) - 4*Il*N*d*dg1*dl*m*m_leg*w*sin(g1 - th) - Il*N*d*dg1^2*l*m*m_leg*w*cos(g1 - th) + 2*It*N*d*dth^2*l*m*m_leg*w*cos(g1 - th))/(4*m*(It*N*l - Il*d*cos(g1 - th) + Il*N*d*cos(g1 - th)));
         (2*GRFz*Il*It*N*sin(g1) - 2*GRFx*Il*It*N*cos(g1) - GRFz*Il*d*m*w*cos(th) - 2*GRFz*Il*d*m_leg*w*cos(th) - GRFx*Il*d*m*w*sin(th) - 2*GRFx*Il*d*m_leg*w*sin(th) - GRFx*Il*N*d^2*m*cos(g1) - 2*Il*N*d*m*t_rb*cos(g1 - th) - 2*Il*N*d*m*t_rf*cos(g1 - th) - 2*GRFx*It*N*l^2*m*cos(g1) + GRFz*Il*N*d^2*m*sin(g1) + 2*GRFz*It*N*l^2*m*sin(g1) - GRFx*Il*N*d^2*m*cos(g1 - 2*th) - 4*Il*It*N*dg1*dl*m - GRFz*Il*N*d^2*m*sin(g1 - 2*th) - 2*Il*d^2*dth^2*m*m_leg*w - GRFz*Il*d*m*w*cos(2*g1 - th) - GRFx*Il*d*m*w*sin(2*g1 - th) - Il*It*N*dg1^2*m*sin(2*g1) - 2*Il*It*N*g*m*sin(g1) - GRFx*d*l^2*m*m_leg*w*sin(th) + Il*It*N*dg1^2*l*m*sin(2*g1) + Il*d*dg1^2*m*m_leg*w*cos(g1 - th) + 2*GRFz*It*N*l*m*w*cos(g1) + 2*GRFz*It*N*l*m_leg*w*cos(g1) + GRFz*Il*N*d*m*w*cos(th) + 2*GRFz*Il*N*d*m_leg*w*cos(th) + 2*GRFx*It*N*l*m*w*sin(g1) + 2*GRFx*It*N*l*m_leg*w*sin(g1) + GRFx*Il*N*d*m*w*sin(th) + 2*GRFx*Il*N*d*m_leg*w*sin(th) - It*N*dg1^2*l*m*m_leg*w + GRFz*d*l^2*m*m_leg*w*cos(2*g1 - th) + GRFx*d*l^2*m*m_leg*w*sin(2*g1 - th) + 2*Il*d*g*m*m_leg*w*cos(th) + Il*d*dg1^2*m*m_leg*w*cos(g1 + th) + 2*Il*N*d^2*dth^2*m*m_leg*w - It*N*dg1^2*l^2*m*m_leg*w + 2*Il*It*N*d*dth^2*m*sin(g1 - th) + GRFz*Il*N*d*m*w*cos(2*g1 - th) + GRFx*Il*N*d*m*w*sin(2*g1 - th) - GRFz*d*l^2*m*m_leg*w*cos(th) + It*N*dg1^2*l^2*m*m_leg*w*cos(2*g1) - Il*N*d*dg1^2*m*m_leg*w*cos(g1 + th) - Il*d*dg1^2*l*m*m_leg*w*cos(g1 + th) + 4*Il*d*dg1*dl*m*m_leg*w*sin(g1 - th) + GRFz*N*d^2*l*m*m_leg*w*cos(g1) + GRFz*N*d*l^2*m*m_leg*w*cos(th) + GRFx*N*d^2*l*m*m_leg*w*sin(g1) + 2*N*d*l*m*m_leg*t_rb*w*sin(g1 - th) + 2*N*d*l*m*m_leg*t_rf*w*sin(g1 - th) + GRFx*N*d*l^2*m*m_leg*w*sin(th) - Il*N*d*dg1^2*m*m_leg*w*cos(g1 - th) - GRFz*N*d^2*l*m*m_leg*w*cos(g1 - 2*th) + GRFx*N*d^2*l*m*m_leg*w*sin(g1 - 2*th) + Il*d*dg1^2*l*m*m_leg*w*cos(g1 - th) - It*N*dg1^2*l*m*m_leg*w*cos(2*g1) - GRFz*N*d*l^2*m*m_leg*w*cos(2*g1 - th) - GRFx*N*d*l^2*m*m_leg*w*sin(2*g1 - th) - 2*It*N*g*l*m*m_leg*w*cos(g1) - 2*Il*N*d*g*m*m_leg*w*cos(th) + Il*N*d*dg1^2*l*m*m_leg*w*cos(g1 + th) - 4*Il*N*d*dg1*dl*m*m_leg*w*sin(g1 - th) - Il*N*d*dg1^2*l*m*m_leg*w*cos(g1 - th) + 2*It*N*d*dth^2*l*m*m_leg*w*cos(g1 - th))/(4*m*(It*N*l - Il*d*cos(g1 - th) + Il*N*d*cos(g1 - th)))];


end

== matlab function deadbeat_running_control/Behavior/Primary and Lateral Behavior/Circular Buffer (Right Foot)/Buffer5 ==
  data: initial_data input; data input; buffer output size=recorded_steps; trigger input; buffer_size input
function buffer  = buffer_data(initial_data, data, trigger, buffer_size)

    persistent buffer_memory
    coder.varsize('buffer_memory',500);
    if isempty(buffer_memory)
        buffer_memory = initial_data;
        if isnan(initial_data(1))
            buffer_memory = [];
        end
    end
    
    if trigger
        buffer_memory = [data; buffer_memory];
        if size(buffer_memory, 1) > buffer_size
            buffer_memory = buffer_memory(1:buffer_size,:);
        end
    end
    
    buffer = buffer_memory;

end

== matlab function deadbeat_running_control/Behavior/Primary and Lateral Behavior/Closed Loop Compensation (Right Foot)/CLOSED LOOP COMPENSATION X FOR VAIRABLE SPEED ==
  data: A_cl input; epsilon input; c input; delta_s_i input; dx_star input; B_cl input; delta_ux output
function delta_ux  = closed_loop_compensation_dxstar...
         (A_cl,epsilon, c, delta_s_i, dx_star, B_cl)
% assume form of delta_s_{i+1} = A_cl*delta_s_i + epsilon +c*dx_star + B_cl*delta_ux
% where delta measures deviation from deadbeat case. solve for
% delta_ux = (-A_cl*delta_s_i-epsilon - c*dxstar)/B_cl to achieve deadbeat
delta_ux = (-A_cl*delta_s_i - epsilon - c*dx_star)/B_cl;

== matlab function deadbeat_running_control/Behavior/Primary and Lateral Behavior/Closed Loop Compensation (Right Foot)/CLOSED LOOP COMPENSATION Y FOR VAIRABLE SPEED ==
  data: A_cl input; epsilon input; c input; delta_s_i input; dx_star input; B_cl input; delta_ux output
function delta_ux  = closed_loop_compensation_dxstar...
         (A_cl,epsilon, c, delta_s_i, dx_star, B_cl)
% assume form of delta_s_{i+1} = A_cl*delta_s_i + epsilon +c*dx_star + B_cl*delta_ux
% where delta measures deviation from deadbeat case. solve for
% delta_ux = (-A_cl*delta_s_i-epsilon - c*dxstar)/B_cl to achieve deadbeat
delta_ux = (-A_cl*delta_s_i - epsilon - c*dx_star)/B_cl;

== matlab function deadbeat_running_control/Behavior/Primary and Lateral Behavior/Closed Loop Compensation (Right Foot)/ESTIMATE CLOSED LOOP ERROR X FOR VARIABLE SPEED ==
  data: dx_land_hist input; A_cl output; delta_ux_hist input; dx_lift_hist input; dx_star_hist input; B_dx_versus_x0 parameter; W_real input; epsilon_0 output; c output; A_cl_nb output; epsilon_0_nb output; c_nb output
function [A_cl, epsilon_0, c, ...
          A_cl_nb, epsilon_0_nb, c_nb] = error_fitting_dxstar...
         (dx_land_hist, delta_ux_hist, dx_lift_hist, dx_star_hist,...
          B_dx_versus_x0, W_real)
% data_length = min([length(dx_lift_hist), filter_length]);
data_length = length(dx_lift_hist);
assert(data_length < 500);
% add fake data
fake_dx_land_err_magnitude = 0.1; fake_dx_star_magnitude = 0.1;
[fgrid_dx_land_err, fgrid_dx_star, fgrid_dx_lift_err] = ...
    meshgrid(fake_dx_land_err_magnitude*[-1 1],fake_dx_star_magnitude*[-1 1],0);
fake_data_length = numel(fgrid_dx_land_err);
fake_dx_land_err = fgrid_dx_land_err(:);
fake_dx_star = fgrid_dx_star(:);
fake_dx_lift_err = fgrid_dx_lift_err(:);
fake_delta_ux = zeros(fake_data_length,1);
% assert(fake_data_length<100);
% assert(filter_length<100);
% fake_dx_land_err = linspace(-0.1, 0.1, fake_data_length)';
% fake_dx_lift_err = zeros(fake_data_length,1);
% fake_delta_ux = zeros(fake_data_length,1);
% fake_dx_star = linspace(-0.25, 0.25, fake_data_length)';
dx_land_err = [reshape(dx_land_hist(1:data_length)-dx_star_hist(1:data_length),...
                       data_length, 1); fake_dx_land_err];
dx_lift_err = [reshape(dx_lift_hist(1:data_length)-dx_star_hist(1:data_length),...
                       data_length, 1); fake_dx_lift_err];
dx_star = [reshape(dx_star_hist(1:data_length), data_length,1); fake_dx_star];
delta_ux = [reshape(delta_ux_hist(1:data_length), data_length, 1); fake_delta_ux];
% weighted least squares
W = diag([W_real*ones(1,data_length), ones(1,fake_data_length)]);
Y = dx_lift_err - B_dx_versus_x0*delta_ux;
X = [dx_land_err, dx_star, ones(data_length+fake_data_length,1)];
% linear regression for s_{i+1}-s0 = A_cl*(s_i-s0) + epsilon_0 + c(s0) + B*delta_u
% solve for Y = X*beta, beta column vector
beta_hat = (X'*W*X)\X'*W*Y;
W_nobias = diag([W_real*ones(1,data_length), 0.001*ones(1,fake_data_length)]);
beta_hat_nobias = (X'*W_nobias*X)\X'*W_nobias*Y;
A_cl = beta_hat(1);
c = beta_hat(2);
epsilon_0 = beta_hat(3);
A_cl_nb = beta_hat_nobias(1);
c_nb = beta_hat_nobias(2);
epsilon_0_nb = beta_hat_nobias(3);

== matlab function deadbeat_running_control/Behavior/Primary and Lateral Behavior/Closed Loop Compensation (Right Foot)/ESTIMATE CLOSED LOOP ERROR Y FOR VARIABLE SPEED ==
  data: dx_land_hist input; A_cl output; delta_ux_hist input; dx_lift_hist input; dx_star_hist input; B_dx_versus_x0 parameter; W_real input; epsilon_0 output; c output; A_cl_nb output; epsilon_0_nb output; c_nb output
function [A_cl, epsilon_0, c, ...
          A_cl_nb, epsilon_0_nb, c_nb] = error_fitting_dxstar...
         (dx_land_hist, delta_ux_hist, dx_lift_hist, dx_star_hist,...
          B_dx_versus_x0, W_real)
% data_length = min([length(dx_lift_hist), filter_length]);
data_length = length(dx_lift_hist);
assert(data_length < 500);
% add fake data
fake_dx_land_err_magnitude = 0.1; fake_dx_star_magnitude = 0.1;
[fgrid_dx_land_err, fgrid_dx_star, fgrid_dx_lift_err] = ...
    meshgrid(fake_dx_land_err_magnitude*[-1 1],fake_dx_star_magnitude*[-1 1],0);
fake_data_length = numel(fgrid_dx_land_err);
fake_dx_land_err = fgrid_dx_land_err(:);
fake_dx_star = fgrid_dx_star(:);
fake_dx_lift_err = fgrid_dx_lift_err(:);
fake_delta_ux = zeros(fake_data_length,1);
% assert(fake_data_length<100);
% assert(filter_length<100);
% fake_dx_land_err = linspace(-0.1, 0.1, fake_data_length)';
% fake_dx_lift_err = zeros(fake_data_length,1);
% fake_delta_ux = zeros(fake_data_length,1);
% fake_dx_star = linspace(-0.25, 0.25, fake_data_length)';
dx_land_err = [reshape(dx_land_hist(1:data_length)-dx_star_hist(1:data_length),...
                       data_length, 1); fake_dx_land_err];
dx_lift_err = [reshape(dx_lift_hist(1:data_length)-dx_star_hist(1:data_length),...
                       data_length, 1); fake_dx_lift_err];
dx_star = [reshape(dx_star_hist(1:data_length), data_length,1); fake_dx_star];
delta_ux = [reshape(delta_ux_hist(1:data_length), data_length, 1); fake_delta_ux];
% weighted least squares
W = diag([W_real*ones(1,data_length), ones(1,fake_data_length)]);
Y = dx_lift_err - B_dx_versus_x0*delta_ux;
X = [dx_land_err, dx_star, ones(data_length+fake_data_length,1)];
% linear regression for s_{i+1}-s0 = A_cl*(s_i-s0) + epsilon_0 + c(s0) + B*delta_u
% solve for Y = X*beta, beta column vector
beta_hat = (X'*W*X)\X'*W*Y;
W_nobias = diag([W_real*ones(1,data_length), 0.001*ones(1,fake_data_length)]);
beta_hat_nobias = (X'*W_nobias*X)\X'*W_nobias*Y;
A_cl = beta_hat(1);
c = beta_hat(2);
epsilon_0 = beta_hat(3);
A_cl_nb = beta_hat_nobias(1);
c_nb = beta_hat_nobias(2);
epsilon_0_nb = beta_hat_nobias(3);

== matlab function deadbeat_running_control/Behavior/Primary and Lateral Behavior/Desired Forward Velocity ==
  data: dx_takeoff input; desired_dx output; desired_forward_velocity input; forward_velocity_target_step parameter
function desired_dx = dx_command(dx_takeoff, desired_forward_velocity, forward_velocity_target_step)
    desired_direction = sign(desired_forward_velocity);
    desired_dx = dx_takeoff + desired_direction*forward_velocity_target_step;
    desired_dx = max(min(desired_dx, abs(desired_forward_velocity)),-abs(desired_forward_velocity));
end
